simulink subsystem "test2slx"  (R2020a)
settings: Solver=VariableStepAuto  StartTime=0.0  StopTime=10.0  RelTol=1e-3
values from neighbouring files (symbols this model uses):
  g = 9.81    [TestingIkRTR.m]    (also in TestingScript.m; TestingScriptRTR.m)
  m2 = 20    [TestingIkRTR.m]    (also in TestingScriptRTR.m)
undefined symbols (not defined in the file or in its folder): I2, m1, p1, p2
settings Model: Creator=ja  LastModifiedBy=ja

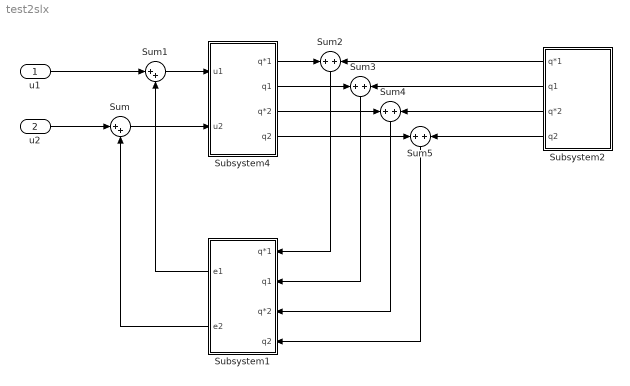
== system test2slx ==
  u1 : Inport
  u2 : Inport  Port=2
  Subsystem1 : Subsystem
  Subsystem2 : Subsystem
  Subsystem4 : Subsystem
  Sum : Sum  Inputs=|++
  Sum1 : Sum  Inputs=|++
  Sum{2..5} (4 alike) : Sum
  wires:
  u2/1 -> Sum/1
  Sum/1 -> Subsystem4/2(u2)
  u1/1 -> Sum1/1
  Sum1/1 -> Subsystem4/1(u1)
  Subsystem4/1(q*1) -> Sum2/1
  Subsystem4/2(q1) -> Sum3/1
  Subsystem4/3(q*2) -> Sum4/1
  Subsystem4/4(q2) -> Sum5/1
  Subsystem2/4(q2) -> Sum5/2
  Subsystem2/3(q*2) -> Sum4/2
  Subsystem2/2(q1) -> Sum3/2
  Subsystem2/1(q*1) -> Sum2/2
  Sum5/1 -> Subsystem1/4(q2)
  Sum4/1 -> Subsystem1/3(q*2)
  Sum3/1 -> Subsystem1/2(q1)
  Sum2/1 -> Subsystem1/1(q*1)
  Subsystem1/1(e1) -> Sum1/2
  Subsystem1/2(e2) -> Sum/2

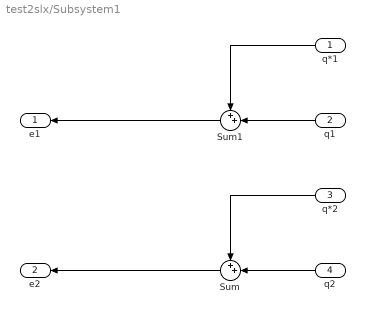
== system test2slx/Subsystem1 ==
  q*1 : Inport
  q1 : Inport  Port=2
  q*2 : Inport  Port=3
  q2 : Inport  Port=4
  Sum : Sum  Inputs=++|
  Sum1 : Sum  Inputs=++|
  e1 : Outport
  e2 : Outport  Port=2
  wires:
  q2/1 -> Sum/2
  Sum/1 -> e2/1
  q*2/1 -> Sum/1
  q1/1 -> Sum1/2
  Sum1/1 -> e1/1
  q*1/1 -> Sum1/1

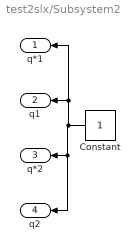
== system test2slx/Subsystem2 ==
  Constant : Constant
  q*1 : Outport
  q1 : Outport  Port=2
  q*2 : Outport  Port=3
  q2 : Outport  Port=4
  wires:
  Constant/1 -> q2/1, q*2/1, q*1/1, q1/1

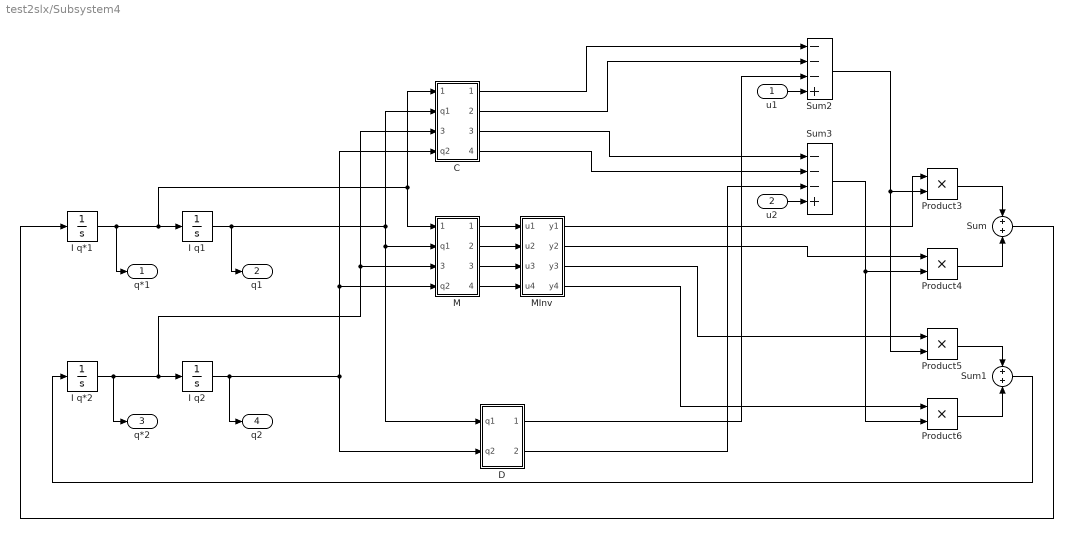
== system test2slx/Subsystem4 ==
  u1 : Inport
  u2 : Inport  Port=2
  C : Subsystem
  D : Subsystem
  I q*1 : Integrator
  I q*2 : Integrator
  I q1 : Integrator
  I q2 : Integrator
  M : Subsystem
  MInv : Subsystem
  Product{3..6} (4 alike) : Product
  Sum : Sum
  Sum1 : Sum
  Sum2 : Sum  Inputs=---+
  Sum3 : Sum  Inputs=---+
  q*1 : Outport
  q1 : Outport  Port=2
  q*2 : Outport  Port=3
  q2 : Outport  Port=4
  wires:
  I q2/1 -> q2/1, C/4(q2), M/4(q2), D/2(q2)
  Sum/1 -> I q*1/1
  MInv/1(y1) -> Product3/1
  M/4(Out4) -> MInv/4(u4)
  D/1(Out1) -> Sum2/3
  I q*1/1 -> q*1/1, I q1/1, C/1(q*1), M/1(q*1)
  Sum1/1 -> I q*2/1
  I q1/1 -> q1/1, D/1(q1), M/2(q1), C/2(q1)
  Product6/1 -> Sum1/2
  Product3/1 -> Sum/1
  I q*2/1 -> q*2/1, M/3(q*2), C/3(q*2), I q2/1
  M/1(Out1) -> MInv/1(u1)
  MInv/4(y4) -> Product6/1
  Product4/1 -> Sum/2
  M/2(Out2) -> MInv/2(u2)
  D/2(Out2) -> Sum3/3
  Sum3/1 -> Product4/2, Product6/2
  Product5/1 -> Sum1/1
  u2/1 -> Sum3/4
  MInv/2(y2) -> Product4/1
  Sum2/1 -> Product5/2, Product3/2
  C/2(Out2) -> Sum2/2
  C/4(Out4) -> Sum3/2
  MInv/3(y3) -> Product5/1
  M/3(Out3) -> MInv/3(u3)
  u1/1 -> Sum2/4
  C/1(Out1) -> Sum2/1
  C/3(Out3) -> Sum3/1

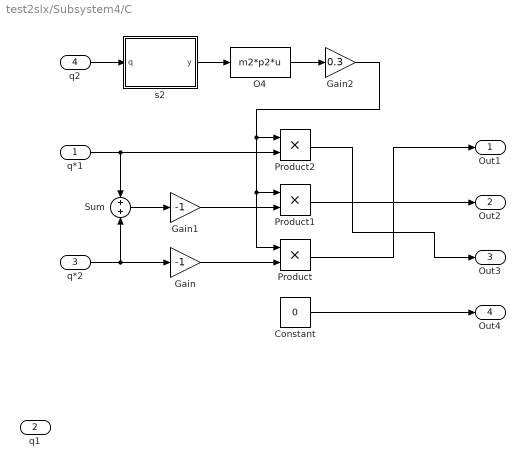
== system test2slx/Subsystem4/C ==
  q*1 : Inport
  q1 : Inport  Port=2
  q*2 : Inport  Port=3
  q2 : Inport  Port=4
  Constant : Constant  Value=0
  Gain : Gain  Gain=-1
  Gain1 : Gain  Gain=-1
  Gain2 : Gain  Gain=0.3
  O4 : Fcn  Expr=m2*p2*u
  Product : Product
  Product1 : Product
  Product2 : Product
  Sum : Sum
  s2 : MATLAB Function  TreatAsAtomicUnit=on
  Out1 : Outport
  Out2 : Outport  Port=2
  Out3 : Outport  Port=3
  Out4 : Outport  Port=4
  wires:
  q*2/1 -> Sum/2, Gain/1
  q2/1 -> s2/1(q)
  q*1/1 -> Product2/2, Sum/1
  s2/1(y) -> O4/1
  O4/1 -> Gain2/1
  Sum/1 -> Gain1/1
  Gain1/1 -> Product1/2
  Gain/1 -> Product/2
  Gain2/1 -> Product/1, Product1/1, Product2/1
  Constant/1 -> Out4/1
  Product/1 -> Out1/1
  Product2/1 -> Out3/1
  Product1/1 -> Out2/1

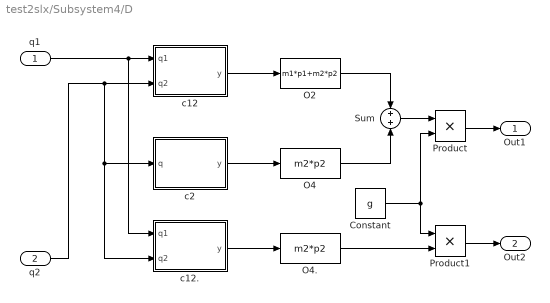
== system test2slx/Subsystem4/D ==
  q1 : Inport
  q2 : Inport  Port=2
  Constant : Constant  Value=g
  O2 : Fcn  Expr=m1*p1+m2*p2
  O4 : Fcn  Expr=m2*p2
  O4. : Fcn  Expr=m2*p2
  Product : Product
  Product1 : Product
  Sum : Sum
  c12 : MATLAB Function  TreatAsAtomicUnit=on
  c12. : MATLAB Function  TreatAsAtomicUnit=on
  c2 : MATLAB Function  TreatAsAtomicUnit=on
  Out1 : Outport
  Out2 : Outport  Port=2
  wires:
  q1/1 -> c12./1(q1), c12/1(q1)
  q2/1 -> c2/1(q), c12./2(q2), c12/2(q2)
  c12/1(y) -> O2/1
  c2/1(y) -> O4/1
  c12./1(y) -> O4./1
  O2/1 -> Sum/1
  O4/1 -> Sum/2
  Product/1 -> Out1/1
  Sum/1 -> Product/1
  Product1/1 -> Out2/1
  Constant/1 -> Product/2, Product1/1
  O4./1 -> Product1/2

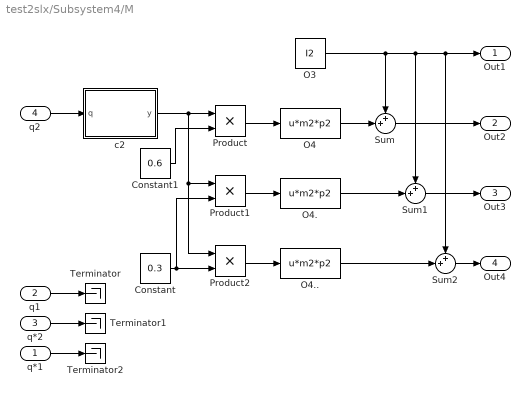
== system test2slx/Subsystem4/M ==
  q*1 : Inport
  q1 : Inport  Port=2
  q*2 : Inport  Port=3
  q2 : Inport  Port=4
  Constant : Constant  Value=0.3
  Constant1 : Constant  Value=0.6
  O3 : Constant  Value=I2
  O4 : Fcn  Expr=u*m2*p2
  O4. : Fcn  Expr=u*m2*p2
  O4.. : Fcn  Expr=u*m2*p2
  Product : Product
  Product1 : Product
  Product2 : Product
  Sum : Sum  Inputs=++|
  Sum1 : Sum  Inputs=++|
  Sum2 : Sum  Inputs=++|
  Terminator : Terminator
  Terminator1 : Terminator
  Terminator2 : Terminator
  c2 : MATLAB Function  TreatAsAtomicUnit=on
  Out1 : Outport
  Out2 : Outport  Port=2
  Out3 : Outport  Port=3
  Out4 : Outport  Port=4
  wires:
  q2/1 -> c2/1(q)
  c2/1(y) -> Product2/1, Product1/1, Product/1
  Constant1/1 -> Product/2
  Constant/1 -> Product1/2, Product2/2
  q1/1 -> Terminator/1
  q*2/1 -> Terminator1/1
  q*1/1 -> Terminator2/1
  Product/1 -> O4/1
  Product2/1 -> O4../1
  Product1/1 -> O4./1
  O4../1 -> Sum2/2
  O4./1 -> Sum1/2
  O4/1 -> Sum/2
  O3/1 -> Out1/1, Sum2/1, Sum1/1, Sum/1
  Sum2/1 -> Out4/1
  Sum/1 -> Out2/1
  Sum1/1 -> Out3/1

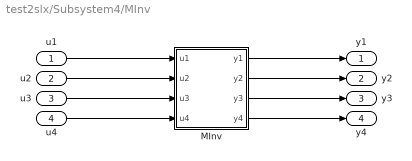
== system test2slx/Subsystem4/MInv ==
  u1 : Inport
  u2 : Inport  Port=2
  u3 : Inport  Port=3
  u4 : Inport  Port=4
  MInv : MATLAB Function  TreatAsAtomicUnit=on
  y1 : Outport
  y2 : Outport  Port=2
  y3 : Outport  Port=3
  y4 : Outport  Port=4
  wires:
  u4/1 -> MInv/4(u4)
  u3/1 -> MInv/3(u3)
  u2/1 -> MInv/2(u2)
  u1/1 -> MInv/1(u1)
  MInv/1(y1) -> y1/1
  MInv/2(y2) -> y2/1
  MInv/3(y3) -> y3/1
  MInv/4(y4) -> y4/1

== matlab function test2slx/Subsystem4/D/c12. ==
  data: q1 input; y output; q2 input
function y = c12(q1, q2)

y = cos(q1+q2);

== matlab function test2slx/Subsystem4/D/c12 ==
  data: q1 input; y output; q2 input
function y = c12(q1, q2)

y = cos(q1+q2);

== matlab function test2slx/Subsystem4/D/c2 ==
  data: q input; y output
function y = c(q)

y = cos(q);

== matlab function test2slx/Subsystem4/M/c2 ==
  data: q input; y output
function y = c(q)

y = cos(q);

== matlab function test2slx/Subsystem4/C/s2 ==
  data: q input; y output
function y = s(q)

y = sin(q);

== matlab function test2slx/Subsystem4/MInv/MInv ==
  data: u1 input; y1 output; u2 input; u3 input; u4 input; y2 output; y3 output; y4 output
function [y1, y2, y3, y4] = c(u1, u2, u3, u4)
y = [u1 u2; u3 u4];
y = inv(y);
y1 = y(1);
y2 = y(2);
y3 = y(3);
y4 = y(4);
